simulink model "bpsk"  (R2016a)
settings: Solver=VariableStepDiscrete  SolverMode=SingleTasking  StartTime=0.0  StopTime=10  RelTol=1e-3
libraries: commdigbbndpm3 x2, commchan3 x1, commsink2 x1, commdigbbndfm2 x1, commrandsrc3 x1
settings Model: Creator=H S  LastModifiedBy=H S
settings DataIOCC: LimitDataPoints=on  SaveOutput=off  SaveTime=off
settings OptimizationCC: BooleanDataType=off  DefaultParameterBehavior=Inlined  LocalBlockOutputs=off
settings DebuggingCC: AlgebraicLoopMsg=error  SingleTaskRateTransMsg=error  AllowSymbolicDim=off
settings ConfigComp: CovModelRefEnable=Off  CovSFcnEnable=off

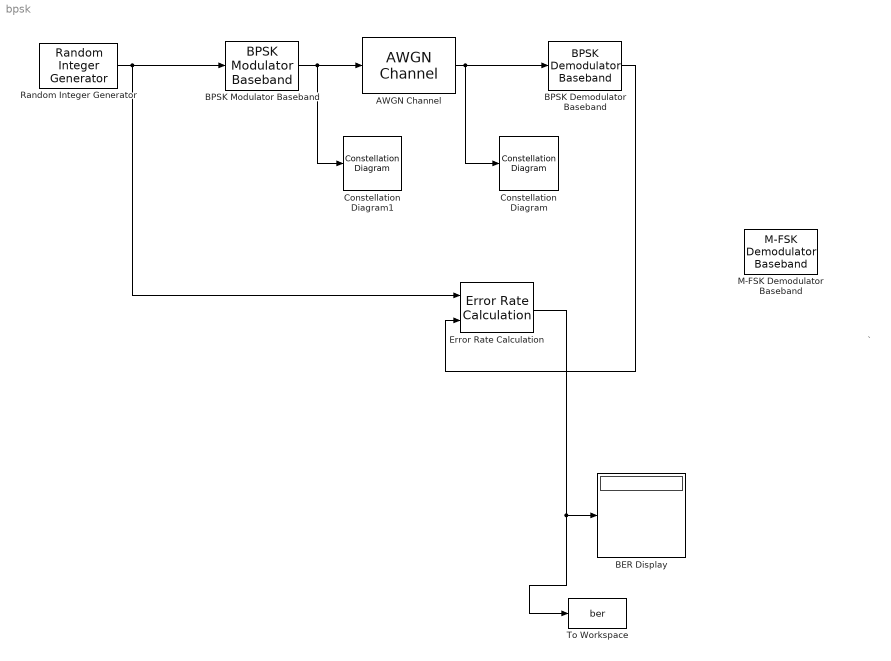
== system bpsk ==
  note: `
  AWGN Channel : commchan3/AWGN Channel  InputProcessing=Columns as channels (frame based)  seed=67  noiseMode="Signal to noise ratio  (Eb/No)"  EbNodB=EbNo  EsNodB=10  SNRdB=10  bitsPerSym=1  Ps=1  Tsym=1  variance=1
  BER Display : Display
  BPSK Demodulator Baseband : commdigbbndpm3/BPSK Demodulator Baseband  DecType=Hard decision  VarSource=Dialog  Variance=1  Ph=0  outDtype=Inherit via internal rule  derotateFactorWordLen=16  derotateFactorDataTypeStr=Inherit: Same word length as input  derotateFactorLastDataTypeStr=Inherit: Same word length as input
  BPSK Modulator Baseband : commdigbbndpm3/BPSK Modulator Baseband  Ph=0  outDtype=double  outWordLen=16  outUDDataType=sfix(16)  outFracLenMode=Best precision  outFracLen=15  outDataTypeStr=double  outLastDataTypeStr=double
  Constellation Diagram : ConstellationDiagram
  Constellation Diagram1 : ConstellationDiagram
  Error Rate Calculation : commsink2/Error Rate Calculation  N=0  st_delay=0  cp_mode=Entire frame  subframe=[]  PMode=Port  WsName=ErrorVec  RsMode2=off  stop=off  numErr=100  maxBits=1e6
  M-FSK Demodulator Baseband : commdigbbndfm2/M-FSK Demodulator Baseband  M=8  OutType=Integer  Dec=Gray  freqSep=6  numSamp=17  RateOptions=Enforce single-rate processing  outDataType=double
  Random Integer Generator : commrandsrc3/Random Integer Generator  SetSize=2  SeedSource=Parameter  Seed=37  SampleTime=1  SamplesPerFrame=100  OutputDataType=uint8  SimulateUsing=Interpreted execution
  To Workspace : ToWorkspace  VariableName=ber  SampleTime=-1
      settings: MaxDataPoints=2  Save2DSignal=2-D array (concatenate along first dimension)
  wires:
  Random Integer Generator/1 -> Error Rate Calculation/1, BPSK Modulator Baseband/1
  AWGN Channel/1 -> Constellation Diagram/1, BPSK Demodulator Baseband/1
  BPSK Demodulator Baseband/1 -> Error Rate Calculation/2
  Error Rate Calculation/1 -> To Workspace/1, BER Display/1
  BPSK Modulator Baseband/1 -> Constellation Diagram1/1, AWGN Channel/1
